simulink model "sampleModel1542_5_sub_sub"  (R2023a)
settings: Solver=VariableStepAuto  StartTime=0.0  StopTime=10.0  RelTol=1e-3
libraries: hdlsllib x6, simulink x5
settings Model: Creator=user1  LastModifiedBy=user1

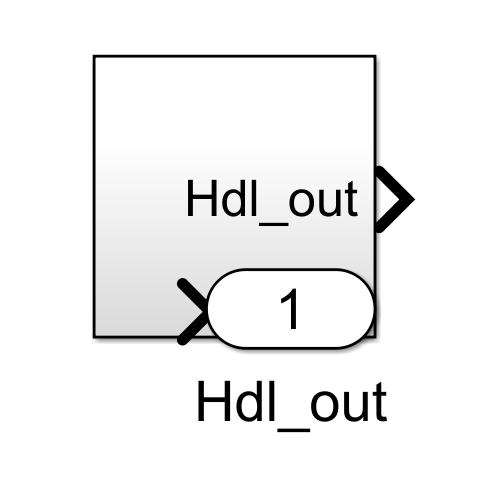
[thumbnail: Simulink's stored preview of the top-level diagram]
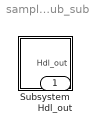
== system sampleModel1542_5_sub_sub ==
  Subsystem : Subsystem
  Hdl_out : Outport  OutDataTypeStr=uint8

== system sampleModel1542_5_sub_sub/Subsystem ==
  Subsystem : Subsystem
  Hdl_out : Outport  OutDataTypeStr=uint8

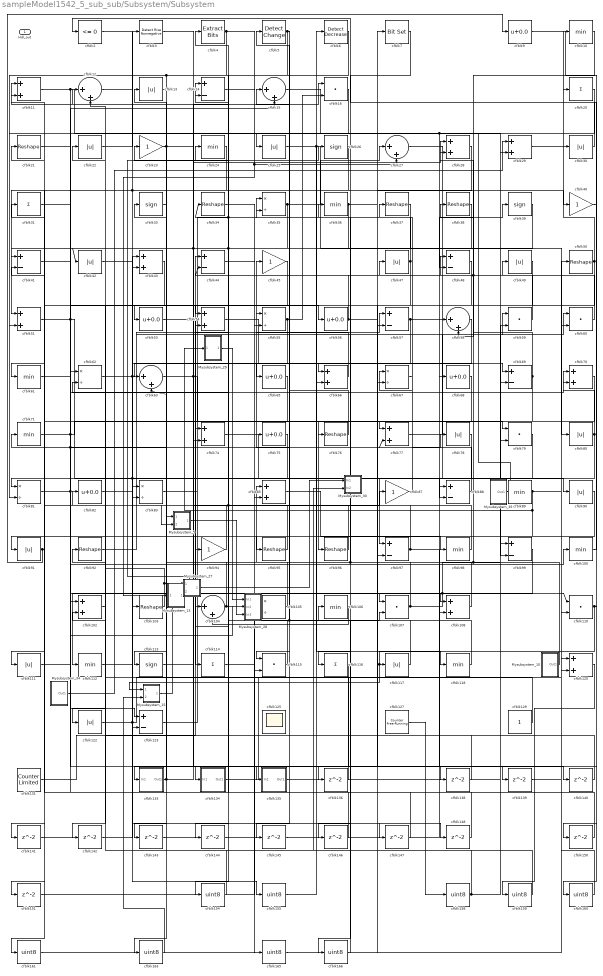
== system sampleModel1542_5_sub_sub/Subsystem/Subsystem ==
  Mysubsystem_10 : Subsystem  TreatAsAtomicUnit=on  RTWFcnName=Mysubsystem_10
      settings: RTWFcnNameOpts=User specified  RTWFileNameOpts=Use function name
  Mysubsystem_13 : Subsystem  TreatAsAtomicUnit=on  RTWFcnName=Mysubsystem_13
      settings: RTWFcnNameOpts=User specified  RTWFileNameOpts=Use function name
  Mysubsystem_15 : Subsystem  TreatAsAtomicUnit=on  RTWFcnName=Mysubsystem_15
      settings: RTWFcnNameOpts=User specified  RTWFileNameOpts=Use function name
  Mysubsystem_27 : Subsystem  TreatAsAtomicUnit=on  RTWFcnName=Mysubsystem_27
      settings: RTWFcnNameOpts=User specified  RTWFileNameOpts=Use function name
  Mysubsystem_28 : Subsystem  TreatAsAtomicUnit=on  RTWFcnName=Mysubsystem_28
      settings: RTWFcnNameOpts=User specified  RTWFileNameOpts=Use function name
  Mysubsystem_29 : Subsystem  TreatAsAtomicUnit=on  RTWFcnName=Mysubsystem_29
      settings: RTWFcnNameOpts=User specified  RTWFileNameOpts=Use function name
  Mysubsystem_30 : Subsystem  TreatAsAtomicUnit=on  RTWFcnName=Mysubsystem_30
      settings: RTWFcnNameOpts=User specified  RTWFileNameOpts=Use function name
  Mysubsystem_34 : Subsystem  TreatAsAtomicUnit=on  RTWFcnName=Mysubsystem_34
      settings: RTWFcnNameOpts=User specified  RTWFileNameOpts=Use function name
  Mysubsystem_35 : Subsystem  TreatAsAtomicUnit=on  RTWFcnName=Mysubsystem_35
      settings: RTWFcnNameOpts=User specified  RTWFileNameOpts=Use function name
  Mysubsystem_5 : Subsystem  TreatAsAtomicUnit=on  RTWFcnName=Mysubsystem_5
      settings: RTWFcnNameOpts=User specified  RTWFileNameOpts=Use function name
  cfblk{10,24,36,61,71,89,98,100,106,112,118} (11 alike) : MinMax  OutDataTypeStr=uint8
  cfblk{11,28..29,43,51,54,66,70,74,77,85,102,108,120} (14 alike) : Sum  OutDataTypeStr=uint8
  cfblk{21,34,37..38,50,76,92,95..96,103} (10 alike) : Reshape
  cfblk{12,15,27,58,63,104} (6 alike) : Sum  Inputs=|++  OutDataTypeStr=uint8
  cfblk{35,55,62,67,81,83,105} (7 alike) : Product  Inputs=*/  OutDataTypeStr=uint8  RndMeth=Zero  SaturateOnIntegerOverflow=on
  cfblk{16,59..60,79,107,110,115} (7 alike) : DotProduct  OutDataTypeStr=uint8
  cfblk{13,22,25,30,42,47,49,78,80,90..91,111,117,122} (14 alike) : Abs  OutDataTypeStr=uint8  SaturateOnIntegerOverflow=off
  cfblk{26,33,39,113} (4 alike) : Signum
  cfblk{20,31,114,116} (4 alike) : Sum  Inputs=+  OutDataTypeStr=uint8
  cfblk{14,41,44,48,57,69,88,97,99,123} (10 alike) : Sum  Inputs=+-  OutDataTypeStr=uint8
  cfblk125 : Scope
      settings: Floating=on
  cfblk127 : hdlsllib/Sources/Counter Free-Running  NumBits=16  tsamp=-1
  cfblk129 : Constant  OutDataTypeStr=uint8  SampleTime=-1
  cfblk131 : hdlsllib/Sources/Counter Limited  uplimit=7  tsamp=-1
  cfblk133 : Subsystem
      settings: LibrarySourceBlock=|
      | hdlsllib/Ports &
      | Subsystems/Subsystem
  cfblk134 : Subsystem
      settings: LibrarySourceBlock=|
      | hdlsllib/Ports &
      | Subsystems/Subsystem
  cfblk135 : Subsystem
      settings: LibrarySourceBlock=|
      | hdlsllib/Ports &
      | Subsystems/Subsystem
  cfblk{136,138..148,150..151} (14 alike) : Delay  SampleTime=1
  cfblk{154..155,158..161,163,165..166} (9 alike) : DataTypeConversion  OutDataTypeStr=uint8  SaturateOnIntegerOverflow=off  RndMeth=Floor
  cfblk2 : hdlsllib/Logic and Bit Operations/Compare To Zero  relop=<=  OutDataTypeStr=uint8
  cfblk{23,40,45,87,94} (5 alike) : Gain  OutDataTypeStr=uint8
  cfblk3 : hdlsllib/Logic and Bit Operations/Detect Rise Nonnegative  vinit=0  OutDataTypeStr=uint8
  cfblk4 : simulink/Logic and Bit Operations/Extract Bits  bitsToExtract=Upper half  numBits=8  bitIdxRange=[0 7]  outScalingMode=Preserve fixed-point scaling
      settings: LibrarySourceBlock=|
      | hdlsllib/Logic and Bit
      | Operations/Extract Bits
  cfblk5 : simulink/Logic and Bit Operations/Detect Change  vinit=0  OutDataTypeStr=uint8
      settings: LibrarySourceBlock=|
      | hdlsllib/Logic and Bit
      | Operations/Detect
      | Change
  cfblk{9,53,56,65,68,75,82} (7 alike) : Bias  Bias=0.0  SaturateOnIntegerOverflow=off
  cfblk6 : simulink/Logic and Bit Operations/Detect Decrease  vinit=0.0  OutDataTypeStr=uint8
      settings: LibrarySourceBlock=|
      | hdlsllib/Logic and Bit
      | Operations/Detect
      | Decrease
  cfblk7 : simulink/Logic and Bit Operations/Bit Set  iBit=0
      settings: LibrarySourceBlock=|
      | hdlsllib/Logic and Bit
      | Operations/Bit Set
  Hdl_out : Outport  OutDataTypeStr=uint8
  wires:
  Mysubsystem_35/1(Out1) -> cfblk74/1, cfblk48/2
  Mysubsystem_34/1(Out1) -> cfblk29/1
  Mysubsystem_27/1(Out1) -> Mysubsystem_30/1(In1)
  Mysubsystem_29/1(Out1) -> Mysubsystem_28/1(In1)
  Mysubsystem_5/1(Out1) -> Mysubsystem_28/3(In3)
  Mysubsystem_15/1(Out1) -> Mysubsystem_27/2(In2)
  cfblk163/1 -> Mysubsystem_15/2(In2)
  Mysubsystem_13/1(Out1) -> cfblk26/1
  Mysubsystem_10/1(Out1) -> cfblk71/1, cfblk28/1
  cfblk166/1 -> cfblk106/1
  cfblk7/1 -> cfblk166/1
  cfblk165/1 -> cfblk7/1
  cfblk114/1 -> cfblk165/1
  cfblk33/1 -> cfblk163/1
  cfblk161/1 -> cfblk120/2
  cfblk160/1 -> cfblk120/1
  cfblk159/1 -> cfblk92/1
  cfblk120/1 -> cfblk159/1
  cfblk158/1 -> Mysubsystem_30/2(In2), cfblk59/2
  cfblk155/1 -> cfblk6/1
  cfblk112/1 -> cfblk155/1
  cfblk154/1 -> cfblk82/1
  cfblk6/1 -> cfblk154/1
  cfblk151/1 -> cfblk105/2
  cfblk65/1 -> cfblk151/1
  cfblk150/1 -> cfblk11/2
  cfblk40/1 -> cfblk150/1
  cfblk148/1 -> cfblk62/1
  cfblk2/1 -> cfblk148/1
  cfblk147/1 -> cfblk104/1
  cfblk44/1 -> cfblk147/1
  cfblk146/1 -> cfblk41/2
  cfblk38/1 -> cfblk146/1
  cfblk145/1 -> cfblk57/2
  cfblk116/1 -> cfblk145/1
  cfblk144/1 -> cfblk58/1
  cfblk143/1 -> cfblk115/2
  cfblk13/1 -> cfblk143/1
  cfblk142/1 -> cfblk83/1
  cfblk45/1 -> cfblk142/1
  cfblk141/1 -> cfblk43/1
  cfblk140/1 -> cfblk12/2
  cfblk139/1 -> cfblk110/2
  cfblk138/1 -> cfblk88/1
  cfblk3/1 -> cfblk138/1
  cfblk136/1 -> cfblk102/2
  cfblk21/1 -> cfblk136/1
  cfblk118/1 -> cfblk23/1
  cfblk78/1 -> cfblk85/2
  cfblk66/1 -> cfblk55/1
  cfblk15/1 -> cfblk99/1
  cfblk98/1 -> cfblk14/1
  cfblk97/1 -> cfblk15/1, cfblk139/1
  cfblk34/1 -> cfblk76/1
  cfblk106/1 -> cfblk104/2
  cfblk4/1 -> cfblk29/2, cfblk81/2
  cfblk74/1 -> cfblk89/1
  cfblk69/1 -> cfblk38/1, cfblk44/2, cfblk116/1
  cfblk57/1 -> cfblk105/1, cfblk39/1
  cfblk59/1 -> cfblk49/1
  cfblk29/1 -> cfblk30/1
  cfblk28/1 -> cfblk123/2, cfblk161/1
  cfblk135/1(Out1) -> cfblk69/2
  cfblk42/1 -> cfblk66/2
  cfblk113/1 -> cfblk16/1
  cfblk5/1 -> cfblk43/2, cfblk63/2, cfblk135/1(In1)
  cfblk31/1 -> cfblk56/1
  cfblk103/1 -> Mysubsystem_27/1(In1), cfblk22/1
  cfblk26/1 -> cfblk41/1
  cfblk100/1 -> cfblk20/1
  cfblk110/1 -> Mysubsystem_15/1(In1), cfblk117/1, cfblk160/1
  cfblk50/1 -> cfblk10/1, cfblk55/2
  cfblk12/1 -> cfblk79/1
  cfblk35/1 -> cfblk63/1, cfblk74/2, cfblk27/1
  cfblk54/1 -> cfblk69/1
  cfblk102/1 -> cfblk122/1
  cfblk61/1 -> cfblk123/1
  cfblk95/1 -> cfblk31/1
  cfblk49/1 -> cfblk61/1
  cfblk23/1 -> Mysubsystem_5/1(In1), cfblk28/2
  cfblk10/1 -> cfblk58/2
  cfblk89/1 -> Mysubsystem_29/1(In1), cfblk99/2, cfblk60/2
  cfblk16/1 -> cfblk54/1
  cfblk122/1 -> cfblk50/1, cfblk78/1
  cfblk63/1 -> cfblk96/1, cfblk108/2
  cfblk39/1 -> cfblk66/1
  cfblk115/1 -> cfblk62/2
  cfblk70/1 -> cfblk94/1
  cfblk56/1 -> cfblk24/1, cfblk140/1
  cfblk22/1 -> cfblk3/1
  cfblk134/1(Out1) -> cfblk68/1
  cfblk68/1 -> cfblk97/2
  cfblk88/1 -> cfblk47/1
  cfblk60/1 -> cfblk48/1
  cfblk67/1 -> cfblk37/1
  cfblk133/1(Out1) -> cfblk13/1, cfblk87/1
  cfblk58/1 -> cfblk115/1
  cfblk76/1 -> cfblk35/2
  cfblk82/1 -> cfblk103/1
  cfblk25/1 -> cfblk80/1, cfblk118/1
  cfblk62/1 -> cfblk57/1, cfblk107/1
  cfblk20/1 -> cfblk51/2
  cfblk51/1 -> Mysubsystem_28/2(In2), cfblk97/1
  cfblk75/1 -> cfblk83/2, cfblk141/1
  cfblk80/1 -> cfblk70/1, cfblk88/2
  cfblk47/1 -> cfblk5/1, cfblk65/1
  cfblk37/1 -> cfblk42/1, cfblk144/1
  cfblk96/1 -> cfblk4/1
  cfblk27/1 -> cfblk90/1
  cfblk81/1 -> cfblk77/2, cfblk15/2, cfblk108/1
  cfblk127/1 -> cfblk158/1
  cfblk107/1 -> cfblk110/1, cfblk79/2, cfblk36/1, cfblk54/2
  cfblk79/1 -> cfblk95/1
  cfblk111/1 -> cfblk100/1
  cfblk83/1 -> cfblk45/1
  cfblk77/1 -> cfblk60/1
  cfblk105/1 -> cfblk11/1
  cfblk36/1 -> cfblk81/1, cfblk40/1
  cfblk48/1 -> cfblk67/2
  cfblk55/1 -> cfblk113/1, cfblk16/2
  cfblk41/1 -> cfblk102/1
  cfblk87/1 -> cfblk67/1
  cfblk9/1 -> cfblk133/1(In1)
  cfblk108/1 -> cfblk85/1
  cfblk94/1 -> cfblk21/1
  cfblk129/1 -> Mysubsystem_5/2(In2), cfblk34/1, cfblk14/2
  cfblk85/1 -> cfblk98/1
  cfblk14/1 -> Mysubsystem_13/1(In1), cfblk27/2
  cfblk117/1 -> cfblk12/1, cfblk75/1
  cfblk71/1 -> cfblk77/1, cfblk70/2
  cfblk99/1 -> cfblk112/1
  cfblk11/1 -> cfblk25/1, cfblk134/1(In1)
  cfblk53/1 -> cfblk114/1
  cfblk43/1 -> cfblk53/1
  cfblk131/1 -> cfblk44/1
  cfblk104/1 -> cfblk33/1, cfblk107/2
  cfblk123/1 -> cfblk35/1
  cfblk91/1 -> cfblk9/1, cfblk111/1
  cfblk24/1 -> cfblk51/1
  cfblk92/1 -> cfblk59/1
  cfblk30/1 -> cfblk2/1
  cfblk90/1 -> cfblk91/1

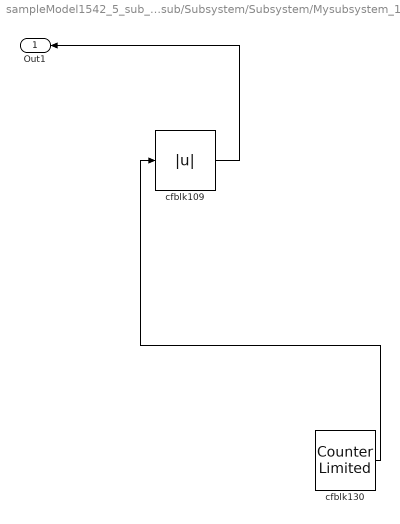
== system sampleModel1542_5_sub_sub/Subsystem/Subsystem/Mysubsystem_10 ==
  cfblk109 : Abs  SaturateOnIntegerOverflow=off
  cfblk130 : hdlsllib/Sources/Counter Limited  uplimit=7  tsamp=-1
  Out1 : Outport
  wires:
  cfblk109/1 -> Out1/1
  cfblk130/1 -> cfblk109/1

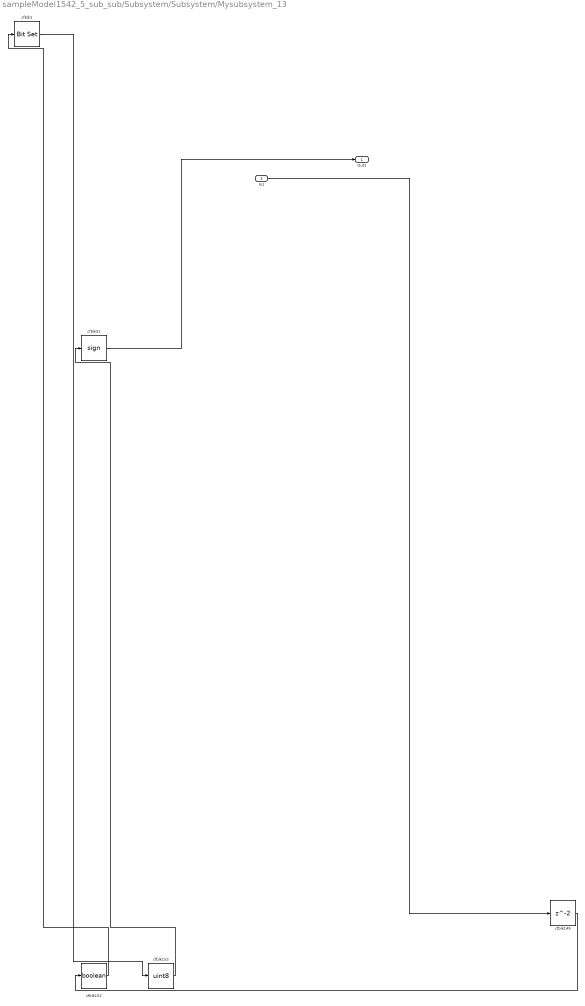
== system sampleModel1542_5_sub_sub/Subsystem/Subsystem/Mysubsystem_13 ==
  In1 : Inport
  cfblk1 : simulink/Logic and Bit Operations/Bit Set  iBit=0
      settings: LibrarySourceBlock=|
      | hdlsllib/Logic and Bit
      | Operations/Bit Set
  cfblk149 : Delay  SampleTime=1
  cfblk152 : DataTypeConversion  OutDataTypeStr=boolean  SaturateOnIntegerOverflow=off  RndMeth=Floor
  cfblk153 : DataTypeConversion  OutDataTypeStr=uint8  SaturateOnIntegerOverflow=off  RndMeth=Floor
  cfblk52 : Signum
  Out1 : Outport
  wires:
  cfblk52/1 -> Out1/1
  cfblk152/1 -> cfblk1/1
  cfblk153/1 -> cfblk52/1
  cfblk1/1 -> cfblk153/1
  cfblk149/1 -> cfblk152/1
  In1/1 -> cfblk149/1

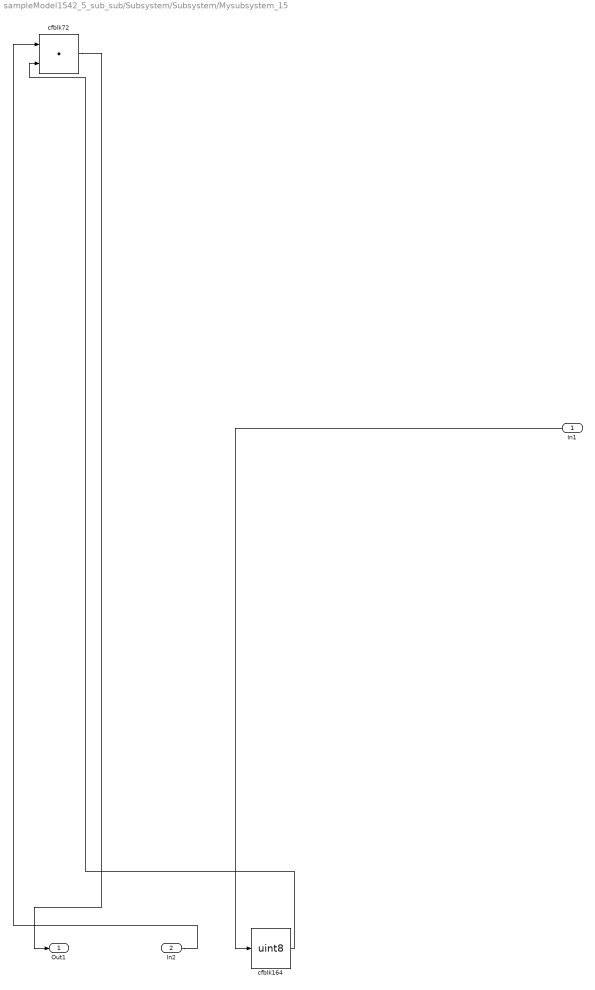
== system sampleModel1542_5_sub_sub/Subsystem/Subsystem/Mysubsystem_15 ==
  In1 : Inport
  In2 : Inport  Port=2
  cfblk164 : DataTypeConversion  OutDataTypeStr=uint8  SaturateOnIntegerOverflow=off  RndMeth=Floor
  cfblk72 : DotProduct  OutDataTypeStr=Inherit: Inherit via internal rule
  Out1 : Outport
  wires:
  cfblk164/1 -> cfblk72/2
  cfblk72/1 -> Out1/1
  In1/1 -> cfblk164/1
  In2/1 -> cfblk72/1

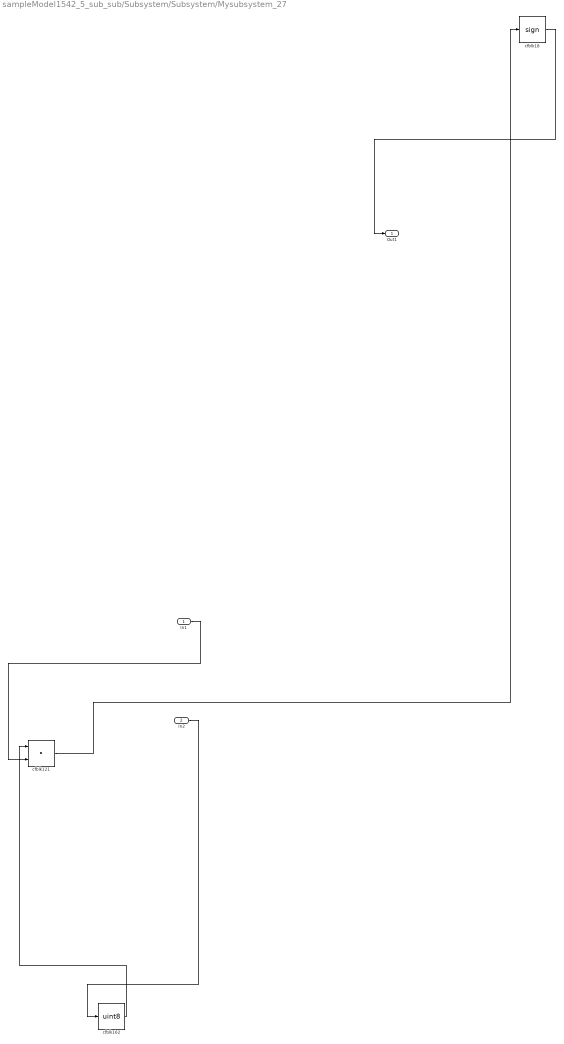
== system sampleModel1542_5_sub_sub/Subsystem/Subsystem/Mysubsystem_27 ==
  In1 : Inport
  In2 : Inport  Port=2
  cfblk121 : DotProduct  OutDataTypeStr=Inherit: Inherit via internal rule
  cfblk162 : DataTypeConversion  OutDataTypeStr=uint8  SaturateOnIntegerOverflow=off  RndMeth=Floor
  cfblk18 : Signum
  Out1 : Outport
  wires:
  cfblk18/1 -> Out1/1
  cfblk121/1 -> cfblk18/1
  In1/1 -> cfblk121/2
  cfblk162/1 -> cfblk121/1
  In2/1 -> cfblk162/1

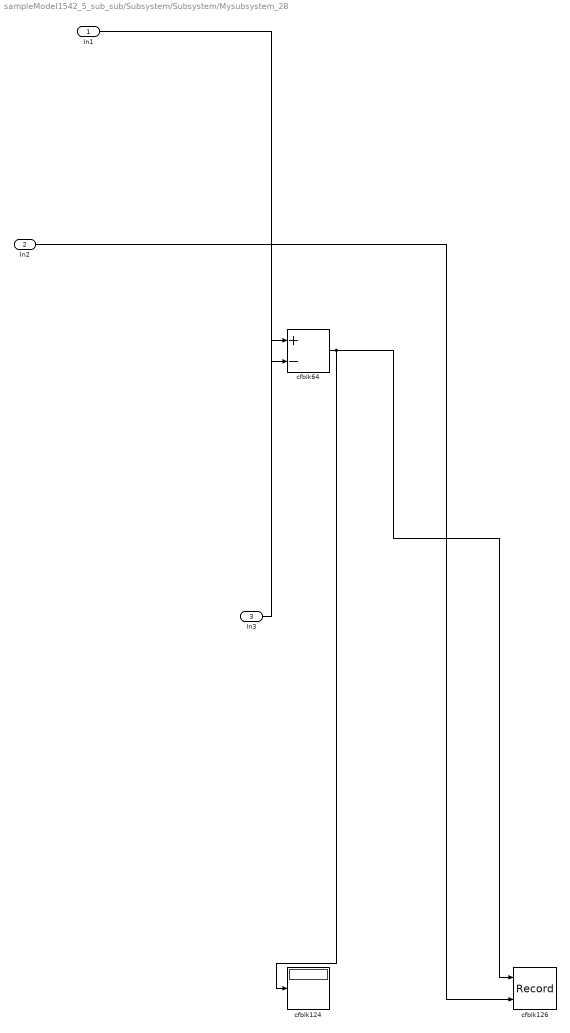
== system sampleModel1542_5_sub_sub/Subsystem/Subsystem/Mysubsystem_28 ==
  In1 : Inport
  In2 : Inport  Port=2
  In3 : Inport  Port=3
  cfblk124 : Display
  cfblk126 : Record  FileSettingsInternal="{\"entries\":[{\"content\":{\"excelSettings\":{\"content\":{},\"type\":\"Streamout.ExcelSettings\"}},\"type\":\"Streamout.FileSettingStorage\",\"uuid\":\"\"}],\"packageUris\":[\"http:\\/\\/schema.mathworks.com\\/mf0\\/streamout_blocks\\/R2020a\"],\"version\":\"1.0\"}"  Layout=[1 1]  SignalsInternal="{\"entries\":[{\"content\":{},\"type\":\"RecordBlkView.InputSignals\",\"uuid\":\"\"}],\"packageUris\":[\"http:\\/\\/schema.mathworks.com\\/mf0\\/streamout_blocks\\/R2020a\"],\"version\":\"1.0\"}"  VisualizationBindings="{\"xyplotplugin\":{\"info\":[{\"series\":[],\"subplotID\":1}]}}"  CompatibilityTag=XY  st=-1
  cfblk64 : Sum  Inputs=+-
  wires:
  cfblk64/1 -> cfblk124/1, cfblk126/1
  In2/1 -> cfblk126/2
  In3/1 -> cfblk64/1
  In1/1 -> cfblk64/2

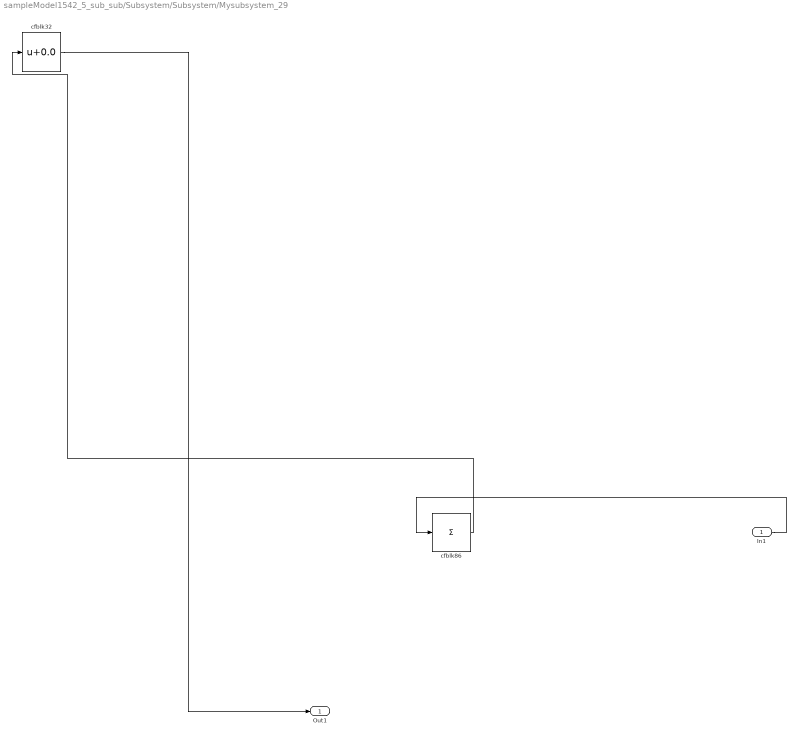
== system sampleModel1542_5_sub_sub/Subsystem/Subsystem/Mysubsystem_29 ==
  In1 : Inport
  cfblk32 : Bias  Bias=0.0  SaturateOnIntegerOverflow=off
  cfblk86 : Sum  Inputs=+
  Out1 : Outport
  wires:
  cfblk86/1 -> cfblk32/1
  cfblk32/1 -> Out1/1
  In1/1 -> cfblk86/1

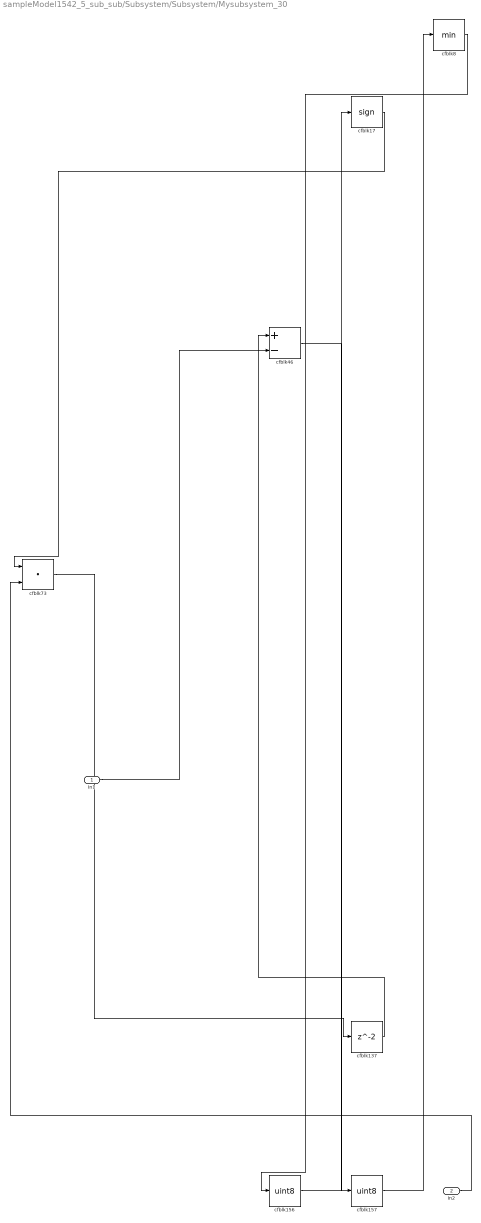
== system sampleModel1542_5_sub_sub/Subsystem/Subsystem/Mysubsystem_30 ==
  In1 : Inport
  In2 : Inport  Port=2
  cfblk137 : Delay  SampleTime=1
  cfblk156 : DataTypeConversion  OutDataTypeStr=uint8  SaturateOnIntegerOverflow=off  RndMeth=Floor
  cfblk157 : DataTypeConversion  OutDataTypeStr=uint8  SaturateOnIntegerOverflow=off  RndMeth=Floor
  cfblk17 : Signum
  cfblk46 : Sum  Inputs=+-
  cfblk73 : DotProduct  OutDataTypeStr=Inherit: Inherit via internal rule
  cfblk8 : MinMax
  wires:
  cfblk157/1 -> cfblk8/1
  cfblk137/1 -> cfblk46/1
  cfblk73/1 -> cfblk137/1
  cfblk17/1 -> cfblk73/1
  cfblk8/1 -> cfblk156/1
  In1/1 -> cfblk46/2
  cfblk156/1 -> cfblk17/1
  cfblk46/1 -> cfblk157/1
  In2/1 -> cfblk73/2

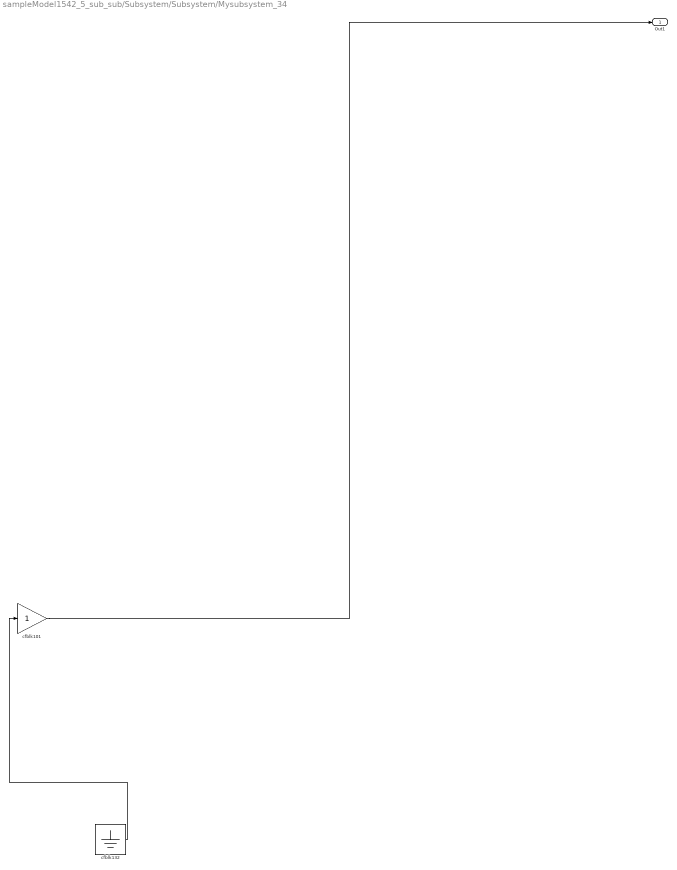
== system sampleModel1542_5_sub_sub/Subsystem/Subsystem/Mysubsystem_34 ==
  cfblk101 : Gain
  cfblk132 : Ground
  Out1 : Outport
  wires:
  cfblk132/1 -> cfblk101/1
  cfblk101/1 -> Out1/1

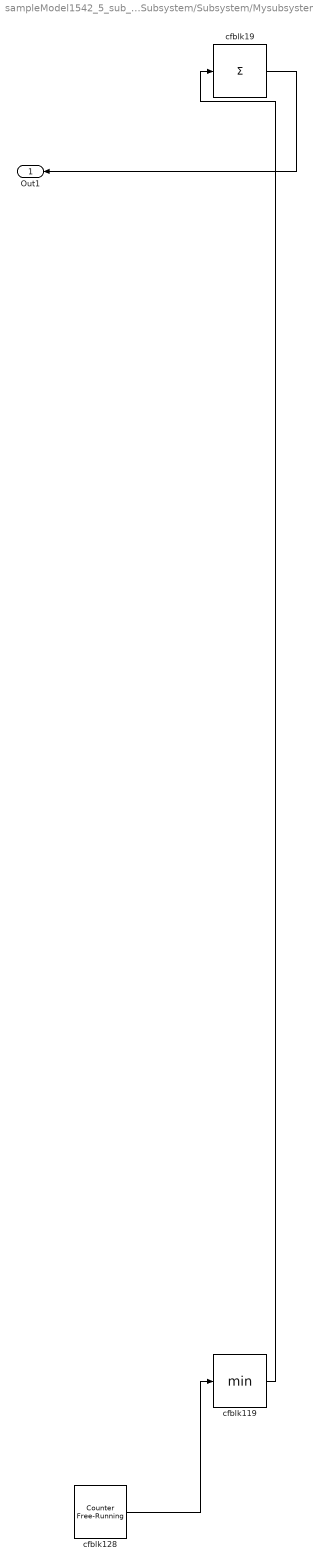
== system sampleModel1542_5_sub_sub/Subsystem/Subsystem/Mysubsystem_35 ==
  cfblk119 : MinMax
  cfblk128 : hdlsllib/Sources/Counter Free-Running  NumBits=16  tsamp=-1
  cfblk19 : Sum  Inputs=+
  Out1 : Outport
  wires:
  cfblk128/1 -> cfblk119/1
  cfblk119/1 -> cfblk19/1
  cfblk19/1 -> Out1/1

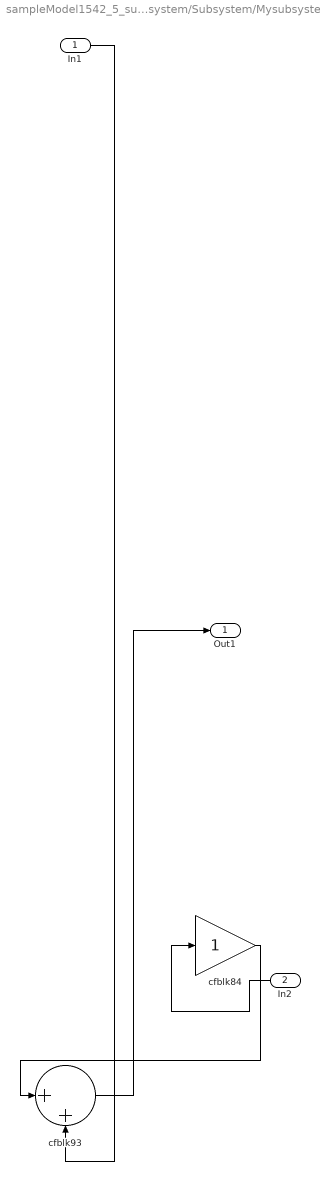
== system sampleModel1542_5_sub_sub/Subsystem/Subsystem/Mysubsystem_5 ==
  In1 : Inport
  In2 : Inport  Port=2
  cfblk84 : Gain
  cfblk93 : Sum  Inputs=|++
  Out1 : Outport
  wires:
  cfblk84/1 -> cfblk93/1
  In2/1 -> cfblk84/1
  In1/1 -> cfblk93/2
  cfblk93/1 -> Out1/1

== system sampleModel1542_5_sub_sub/Subsystem/Subsystem/cfblk133 ==
  In1 : Inport
  Out1 : Outport
  wires:
  In1/1 -> Out1/1

== system sampleModel1542_5_sub_sub/Subsystem/Subsystem/cfblk134 ==
  In1 : Inport
  Out1 : Outport
  wires:
  In1/1 -> Out1/1

== system sampleModel1542_5_sub_sub/Subsystem/Subsystem/cfblk135 ==
  In1 : Inport
  Out1 : Outport
  wires:
  In1/1 -> Out1/1
